simulink model "testeCeq"  (R2017a)
settings: Solver=VariableStepAuto  StartTime=0.0  StopTime=150  RelTol=1e-3
values from neighbouring files (symbols this model uses):
  Ceq = NumCeq/DenCeq    [Item3PSF.m]    (also in item3_PSF_comK.m = minreal((C_d*Fr)/(1+ C_d*Gu_d*(1-Fr*z^-40)), 1e-2); psfRapido.m)
  Fn = F_d/Fr    [Item3PSF.m]    (also in psfRapido.m = 1/Fr)
  Ts = t_5/20    (= 0.075)    [Item3PSF.m]    (also in item3_PSF_comK.m; psfRapido.m; robustezPSF.m)
settings Model: Creator=julia  LastModifiedBy=julia

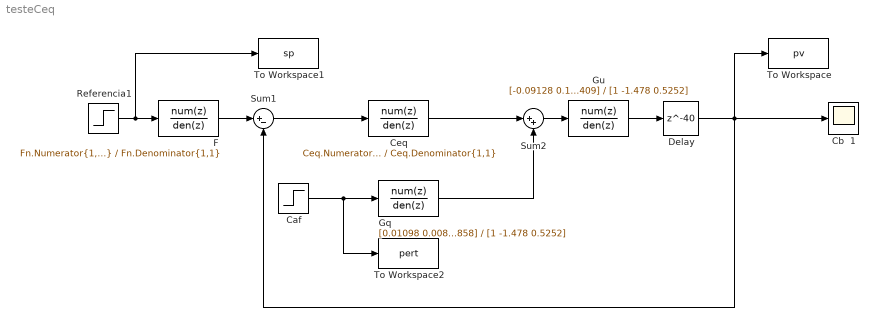
== system testeCeq ==
  Caf : Step  Time=40  After=0.1  SampleTime=Ts
  Cb  1 : Scope
  Ceq : DiscreteTransferFcn  Numerator=Ceq.Numerator{1,1}  Denominator=Ceq.Denominator{1,1}  SampleTime=Ts
  Delay : Delay  DelayLength=40  InitialCondition=0
  F : DiscreteTransferFcn  Numerator=Fn.Numerator{1,1}  Denominator=Fn.Denominator{1,1}  SampleTime=Ts
  Gq : DiscreteTransferFcn  Numerator=[0.01098 0.008858]  Denominator=[1 -1.478 0.5252]  SampleTime=Ts
  Gu : DiscreteTransferFcn  Numerator=[-0.09128 0.1409]  Denominator=[1 -1.478 0.5252]  SampleTime=Ts
  Referencia1 : Step  Time=0  SampleTime=Ts
  Sum1 : Sum  Inputs=|+-
  Sum2 : Sum  Inputs=|++
  To Workspace : ToWorkspace  VariableName=pv  SaveFormat=Timeseries  SampleTime=-1
  To Workspace1 : ToWorkspace  VariableName=sp  SaveFormat=Timeseries  SampleTime=-1
  To Workspace2 : ToWorkspace  VariableName=pert  SaveFormat=Timeseries  SampleTime=-1
  wires:
  Sum1/1 -> Ceq/1
  Ceq/1 -> Sum2/1
  Sum2/1 -> Gu/1
  Caf/1 -> To Workspace2/1, Gq/1
  Gq/1 -> Sum2/2
  Gu/1 -> Delay/1
  Delay/1 -> Sum1/2, To Workspace/1, Cb  1/1
  F/1 -> Sum1/1
  Referencia1/1 -> To Workspace1/1, F/1
